simulink model "Continues_motor_control_v9_tensiontest"  (R2025b)
settings: Solver=FixedStepAuto  StartTime=0.0  StopTime=Duration_time  FixedStep=T_sample  RelTol=1e-3  EnableMultiTasking=on
undefined symbols (not defined in the file or in its folder): bias, cyclenum, Ki, Kp, N_finish, N_start, Potent_gain, T, T_sample, v_0, Voltage
libraries: slrealtimeloglib x4, speedgoatlib_IO131 x3, simulink x1
settings Model: Creator=User  LastModifiedBy=paola
settings SolverCC: ConcurrentTasks=on  AlgebraicLoopSolver=TrustRegion  PositivePriorityOrder=on  AutoInsertRateTranBlk=on  InsertRTBMode=Never (minimum delay)
settings DataIOCC: SaveFormat=Array  SaveState=on  SignalLoggingName=logsOut
settings OptimizationCC: BlockReduction=off  BooleanDataType=off  OptimizeBlockIOStorage=off  BufferReuse=off  ReuseModelBlockBuffer=off  GlobalBufferReuse=off  ExpressionFolding=off  LocalBlockOutputs=off  InitFltsAndDblsToZero=on  OptimizeDataStoreBuffers=off  BusAssignmentInplaceUpdate=off
settings DebuggingCC: SaveWithParameterizedLinksMsg=none  UnderspecifiedInitializationDetection=Classic  MergeDetectMultiDrivingBlocksExec=none  CheckExecutionContextPreStartOutputMsg=on  SignalResolutionControl=TryResolveAllWithWarning  TasksWithSamePriorityMsg=none  UnconnectedInputMsg=warning  UnconnectedOutputMsg=warning  UnconnectedLineMsg=warning  SFUnexpectedBacktrackingDiag=warning  SFNoUnconditionalDefaultTransitionDiag=warning  SFExecutionAtInitializationDiag=none  ArithmeticOperatorsInVariantConditions=warning
settings HardwareCC: ProdBitPerLong=64.0  ProdLongLongMode=on  ProdHWDeviceType=Intel->x86-64 (Linux 64)
settings ModelReferenceCC: EnableRefExpFcnMdlSchedulingChecks=on  PropagateSignalLabelsOutOfModel=off
settings SFSimCC: SimUseLocalCustomCode=off  SimTargetLang=C++  SimDLTargetLibrary=mkl-dnn
settings RTWCC: SystemTargetFile=speedgoat.tlc  TemplateMakefile=slrealtime_default_tmf  RTWUseLocalCustomCode=off  Toolchain=Simulink Real-Time Toolchain  BuildConfiguration=Faster Runs  CodeExecutionProfiling=on  TargetLang=C++  GPUComputeCapability=3.5  DLArmComputeVersion=19.05  Description=Speedgoat Real-Time Target Machine
settings CodeAppCC: StateflowObjectComments=on
settings SimulinkRealTimeTargetCC: SLRTFileLogMaxRuns=1.0  ExtModeMaxTrigDuration=10.0  ExtModeStaticAllocSize=1000000.0  ExtModeTransport=0.0  MultiwordLength=2048.0  DynamicStringBufferSize=256.0  PreserveMATLABNamespacesInGeneratedCode=on  SubcomponentCodeInterfacePackaging=Reusable function  InstructionSetFMA=off  LogToMDFFile=off
settings ConfigComp: CovMetricSettings=dw  CovSaveCumulativeToWorkspaceVar=on  CovSaveSingleToWorkspaceVar=on  CovExternalEMLEnable=off  CovSFcnEnable=off

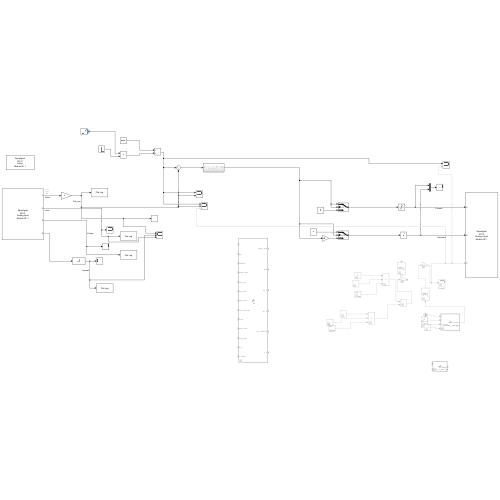
[thumbnail: Simulink's stored preview of the top-level diagram]
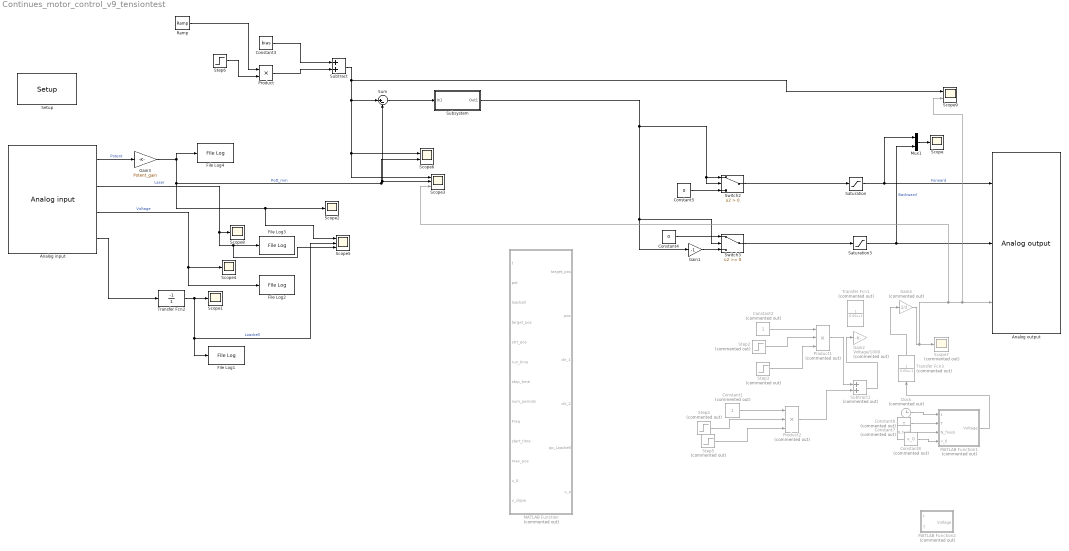
== system Continues_motor_control_v9_tensiontest ==
  "Analog input " : speedgoatlib_IO131/Analog input   parModuleId=1  parSampleTime=-1  parPciSlot=-1  parRange=+-10V  parOversampling=None  parChannels=[1 2 3 4]  parContinuousSampling=off  parDmaEn=off  parDmaChannels=All  parDmaConversionTime=100  parDmaFrameSize=128  parBoardType=131  parIsInitialized=on
      settings: SourceProductName=IO131
  "Analog output " : speedgoatlib_IO131/Analog output   parModuleId=1  parSampleTime=-1  parPciSlot=-1  parRange=+-10V  parChannels=[5 6 7]  parInitValues=[0 0 0]  parResetValues=[1 1 1]  parDmaChannels=All  parDmaEn=off  parDmaClkSrc=2  parDmaConversionTime=100  parDmaFrameSize=128  parBoardType=131  parDoInterrupt=on  parLatency=As small as possible  parIsInitialized=on
      settings: SourceProductName=IO131
  Clock : Clock  Commented=on
  Constant1 : Constant  Commented=on
  Constant2 : Constant  Commented=on
  Constant3 : Constant  Value=bias
  Constant4 : Constant  Value=0
  Constant5 : Constant  Value=0
  Constant6 : Constant  Commented=on  Value=T
  Constant7 : Constant  Commented=on  Value=N_finish
  Constant8 : Constant  Commented=on  Value=v_0
  File Log{1..4} (4 alike) : slrealtimeloglib/File Log  decimation=1  inputProcessing=Elements as channels (sample based)
  Gain1 : Gain  Gain=-1
  Gain2 : Gain  Commented=on  Gain=Voltage/1000
  Gain3 : Gain  Gain=Potent_gain
  Gain4 : Gain  Commented=on  Gain=2/3
  MATLAB Function : MATLAB Function  Commented=on  TreatAsAtomicUnit=on  SystemSampleTime=1/20000
  MATLAB Function1 : MATLAB Function  Commented=on  TreatAsAtomicUnit=on
  MATLAB Function2 : MATLAB Function  Commented=on  TreatAsAtomicUnit=on
  Mux1 : Mux  Inputs=2
  Product : Product
  Product1 : Product  Commented=on  Inputs=3
  Product2 : Product  Commented=on  Inputs=3
  Ramp : simulink/Sources/Ramp  slope=0.5  start=3*T  InitialOutput=0
  Saturation : Saturate  UpperLimit=5  LowerLimit=0
  Saturation3 : Saturate  UpperLimit=5  LowerLimit=0
  Scope{,1..2,4,8} (5 alike) : Scope
      Scope settings: ActiveDisplayYMinimum=-0.62499999999999989  ActiveDisplayYMaximum=5.625
      Scope1 settings: ActiveDisplayYMinimum=-0.40301743822598  ActiveDisplayYMaximum=-0.37430870981834546  DataLoggingVariableName=ScopeData2
      Scope2 settings: ActiveDisplayYMinimum=47.04763  ActiveDisplayYMaximum=48.80097  DataLoggingVariableName=ScopeData3
      Scope4 settings: ActiveDisplayYMinimum=-3.531161659188478  ActiveDisplayYMaximum=3.4859297139005889  DataLoggingVariableName=ScopeData5
      Scope8 settings: ActiveDisplayYMinimum=2.5736629282063022  ActiveDisplayYMaximum=3.1252765697718781  DataLoggingVariableName=ScopeData7
  Scope3 : Scope  NumInputPorts=3
      settings: ActiveDisplayYMinimum=61.500028125  ActiveDisplayYMaximum=146.499996875  DataLoggingVariableName=ScopeData4
  Scope5 : Scope  NumInputPorts=3
      settings: ActiveDisplayYMinimum=34.92623025864043  ActiveDisplayYMaximum=149.50569161516748
  Scope6 : Scope  NumInputPorts=2
      settings: ActiveDisplayYMinimum=-16.874999999999996  ActiveDisplayYMaximum=151.875  DataLoggingVariableName=ScopeData6
  Scope7 : Scope  Commented=on
      settings: ActiveDisplayYMinimum=-4.9999999896942331  ActiveDisplayYMaximum=4.9999999896942331  DataLoggingVariableName=ScopeData2
  Scope9 : Scope  NumInputPorts=2
      settings: ActiveDisplayYMinimum=57.0000140625  ActiveDisplayYMaximum=146.9999984375  DataLoggingVariableName=ScopeData8
  "Setup " : speedgoatlib_IO131/Setup   parPciSlot=-1  parModuleId=1  parTriggerInitiator=Independent  parAdChannels=1:4  parAdRange=+-10V  parAdOversampling=None  parAdContinuousSampling=off  parAdDmaEn=off  parAdDisableCheck=off  parAdDmaChannels=All  parAdSampleClock=1e3  parAdDmaFrameSize=128  parAdSampleTime=-1  parDaChannels=5:7  parDaRange=+-10V  parDaInitValues=0  parDaResetValues=1  parDaDmaEn=off  parDaDisableCheck=off  parDaDmaChannels=All  parLatency=As small as possible  parDaSampleClock=1e3  parClockLocked=on  parDaDmaFrameSize=128  parDaSampleTime=-1  parBoardType=131  parForceRefresh=[]
      settings: SourceProductName=IO131
  Step2 : Step  Commented=on  Time=(N_start-0.25)*T  SampleTime=T_sample
  Step3 : Step  Commented=on  Time=(cyclenum+0.25)*T  Before=1  After=0  SampleTime=T_sample
  Step4 : Step  Commented=on  Time=(2*cyclenum+0.25)*T  SampleTime=T_sample
  Step5 : Step  Commented=on  Time=(cyclenum+0.25)*T  Before=1  After=0  SampleTime=T_sample
  Step6 : Step  Time=N_finish*T  Before=1  After=0  SampleTime=T_sample
  Subsystem : Subsystem
  Subtract : Sum
  Subtract1 : Sum  Commented=on
  Sum : Sum  Inputs=|+-
  Switch2 : Switch  Criteria=u2 > Threshold  SaturateOnIntegerOverflow=off  InputSameDT=off
  Switch3 : Switch  SaturateOnIntegerOverflow=off  InputSameDT=off
  Transfer Fcn1 : TransferFcn  Commented=on  Denominator=[0.05 1]
  Transfer Fcn2 : TransferFcn  Numerator=[-1]  Denominator=[1 ]
  Transfer Fcn3 : TransferFcn  Commented=on  Denominator=[0.05 1]
  wires:
  "Analog input "/4 -> Transfer Fcn2/1
  Constant5/1 -> Switch2/3
  Transfer Fcn2/1 -> Scope5/2, File Log1/1, Scope1/1  "Loadcell"
  Gain3/1 -> Scope6/2, Scope3/2, Sum/2, Scope5/1, Scope2/1, File Log4/1  "Pott_mm"
  Saturation/1 -> "Analog output "/1, Mux1/1  "Forward"
  Gain1/1 -> Switch3/3
  Subsystem/1(Out1) -> Gain1/1, Switch3/2, Switch2/1, Switch2/2
  Constant4/1 -> Switch3/1
  Switch3/1 -> Saturation3/1
  "Analog input "/1 -> Gain3/1  "Potent"
  Sum/1 -> Subsystem/1(In1)
  Mux1/1 -> Scope/1
  Switch2/1 -> Saturation/1
  Saturation3/1 -> "Analog output "/2, Mux1/2  "Backward"
  "Analog input "/3 -> File Log2/1, Scope4/1  "Voltage"
  Step6/1 -> Product/2
  Ramp/1 -> Product/1
  Constant2/1 -> Product1/1
  Transfer Fcn3/1 -> Gain4/1
  Step2/1 -> Product1/2
  Step3/1 -> Product1/3
  Product1/1 -> Subtract1/1
  Product2/1 -> Subtract1/2
  Constant1/1 -> Product2/1
  Step4/1 -> Product2/2
  Step5/1 -> Product2/3
  Subtract1/1 -> Gain2/1
  Clock/1 -> MATLAB Function1/1(t)
  Constant6/1 -> MATLAB Function1/2(T)
  "Analog input "/2 -> Scope5/3, File Log3/1, Scope8/1  "Laser"
  MATLAB Function1/1(Voltage) -> Transfer Fcn3/1
  Product/1 -> Subtract/2
  Constant3/1 -> Subtract/1
  Subtract/1 -> Scope3/1, Scope6/1, Sum/1, Scope9/1
  Gain4/1 -> Scope3/3, Scope9/2, "Analog output "/3, Scope7/1
  Constant7/1 -> MATLAB Function1/3(N_finish)
  Constant8/1 -> MATLAB Function1/4(v_0)

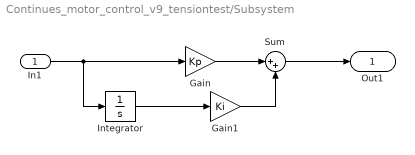
== system Continues_motor_control_v9_tensiontest/Subsystem ==
  In1 : Inport
  Gain : Gain  Gain=Kp
  Gain1 : Gain  Gain=Ki
  Integrator : Integrator
  Sum : Sum  Inputs=|++
  Out1 : Outport
  wires:
  In1/1 -> Integrator/1, Gain/1
  Sum/1 -> Out1/1
  Gain/1 -> Sum/1
  Gain1/1 -> Sum/2
  Integrator/1 -> Gain1/1

== matlab function Continues_motor_control_v9_tensiontest/MATLAB Function1 ==
  data: t input; Voltage output; T input; N_finish input; v_0 input
function Voltage = generate_voltage(t, T, N_finish, v_0)
% Generates a voltage waveform with:
% - 3T initial rest (0 V)
% - N cycles of pattern [0, +2, 0, -2]
% - 1T final rest (0 V)
%
% t : current time
% T : one cycle duration
% N : number of active cycles

   % total_time = Initial a*T rest + applying voltage_time*T + final resting*T;  % total signal duration
     total_time = (N_finish-1)*T;

    if t < 1*T
        % Initial 3T rest
        Voltage = 0;

    elseif t < (1 + (N_finish-2))*T
        % Active part (N cycles)
        active_time = t - 2*T;   % time since the active section started
        phase = mod(active_time, T);
        quarter = T / 4;

        if phase < quarter
            Voltage = 0;
        elseif phase < 2*quarter
            Voltage = v_0;
        elseif phase < 3*quarter
            Voltage = 0;
        elseif phase < 4*quarter
            Voltage = -v_0;
        else
            Voltage = 0;
        end

    elseif t < total_time
        % Final 1T rest
        Voltage = 0;

    else
        % After everything
        Voltage = 0;
    end
end

== matlab function Continues_motor_control_v9_tensiontest/MATLAB Function ==
  data: target_pos output; t input; pot input; loadcell input; pos output; dir_1 output; target_pos input; dir_2 output; strt_pos input; run_time input; stop_time input; num_periods input; Freq input; start_time input; max_pos input; v_0 input; v_slope input; pp_Loadcell output; v_o output
function [target_pos,pos,dir_1,dir_2,pp_Loadcell, v_o] = fcn(t,pot,loadcell,target_pos,strt_pos,run_time,stop_time,num_periods,Freq,start_time,max_pos,v_0,v_slope)

persistent strt_pos_th I;

if isempty(strt_pos_th)
 strt_pos_th = strt_pos;

 I=0;
 last_err=0;
end

v_o=0;
v=0;

loadcell_thr = -0.3; % In N

% cal_loadcell = 2.7384;%0.9936;%-1.6080;
% offset_loadcell =   0.2727; %0.2868;%0.1759;
% 
% cal_weight = 0.399*10;
% pp_Loadcell = (loadcell - offset_loadcell).*(cal_weight/(cal_loadcell-offset_loadcell));
C_1 = 1.5635;
pp_Loadcell = (loadcell-0.3058)*C_1 ;


if(t>(run_time-stop_time))
    v = 0;
elseif(t>(start_time-0.1))
    v = v_0;

    
    if(pp_Loadcell>loadcell_thr)
        target_pos = (strt_pos-3)+5/start_time.*t;
        strt_pos_th = target_pos;
    else
        target_pos = strt_pos_th;
    end

end

%persistent pwm_val;

%if isempty(X)
%  X = [0 0 0]; 
%  P =  diag([10000,10000,10000]);
%end

% if(t>(run_time-stop_time))
%     target_pos=strt_pos-3;
% end

dir_1 = 0;
dir_2 = 0;



v_o=v/1000;

end

== matlab function Continues_motor_control_v9_tensiontest/MATLAB Function2 ==
  data: t input; Voltage output; T input
function Voltage = generate_voltage(t, T)
% t: current time
% T: time period

    if t < (T)
        Voltage = 0;
    elseif t < (T+T*1/4)
        Voltage = 2;
    elseif t < (T+T*1/2)
        Voltage = 0;
    elseif t < (T+T*3/4)
        Voltage = -2;
    elseif t < (2*T)
        Voltage = 0;
    elseif t < (2*T+T*1/4)
        Voltage = 2;
    elseif t < (2*T+T*1/2)
        Voltage = 0;
    elseif t < (2*T+T*3/4)
        Voltage = -2;
    elseif t < (3*T)
        Voltage = 0;
    elseif t < (3*T+T*1/4)
        Voltage = 2;
    elseif t < (3*T+T*1/2)
        Voltage = 0;
    elseif t < (3*T+T*3/4)
        Voltage = -2;
    elseif t < (4*T)
        Voltage = 0;
    elseif t < (4*T+T*1/4)
        Voltage = 2;
    elseif t < (4*T+T*1/2)
        Voltage = 0;
    elseif t < (4*T+T*3/4)
        Voltage = -2;
    elseif t < (5*T)
        Voltage = 0;
    elseif t < (5*T+T*1/4)
        Voltage = 2;
    elseif t < (5*T+T*1/2)
        Voltage = 0;
    elseif t < (5*T+T*3/4)
        Voltage = -2;
    elseif t < (6*T)
        Voltage = 0;
    elseif t < (6*T+T*1/4)
        Voltage = 2; 
    elseif t < (6*T+T*1/2)
        Voltage = 0;
    elseif t < (6*T+T*3/4)
        Voltage = -2;
    elseif t < (7*T)
        Voltage = 0;
    elseif t < (7*T+T*1/4)
        Voltage = 2;
    elseif t < (7*T+T*1/2)
        Voltage = 0;
    elseif t < (7*T+T*3/4)
        Voltage = -2;
    elseif t < (8*T)
        Voltage = 0;
    elseif t < (8*T+T*1/4)
        Voltage = 2;
    elseif t < (8*T+T*1/2)
        Voltage = 0;
    elseif t < (8*T+T*3/4)
        Voltage = -2;
    elseif t < (9*T)
        Voltage = 0;
    elseif t < (9*T+T*1/4)
        Voltage = 2;
    elseif t < (9*T+T*1/2)
        Voltage = 0;
    elseif t < (9*T+T*3/4)
        Voltage = -2;
    elseif t < (10*T)
        Voltage = 0;
    elseif t < (10*T+T*1/4)
        Voltage = 2;
    elseif t < (10*T+T*1/2)
        Voltage = 0;
    elseif t < (10*T+T*3/4)
        Voltage = -2;
    elseif t < (11*T)
        Voltage = 0;
    elseif t < (11*T+T*1/4)
        Voltage = 2;
    elseif t < (11*T+T*1/2)
        Voltage = 0;
    elseif t < (11*T+T*3/4)
        Voltage = -2;
    elseif t < (12*T)
        Voltage = 0;
    elseif t < (12*T+T*1/4)
        Voltage = 2;
    elseif t < (12*T+T*1/2)
        Voltage = 0;
    elseif t < (12*T+T*3/4)
        Voltage = -2;
    elseif t < (13*T)
        Voltage = 0;
    elseif t < (13*T+T*1/4)
        Voltage = 2;
    elseif t < (13*T+T*1/2)
        Voltage = 0;
    elseif t < (13*T+T*3/4)
        Voltage = -2;
    elseif t < (14*T)
        Voltage = 0;
    elseif t < (14*T+T*1/4)
        Voltage = 2;
    elseif t < (14*T+T*1/2)
        Voltage = 0;
    elseif t < (14*T+T*3/4)
        Voltage = -2;
    elseif t < (15*T)
        Voltage = 0;
    elseif t < (15*T+T*1/4)
        Voltage = 2;
    elseif t < (15*T+T*1/2)
        Voltage = 0;
    elseif t < (15*T+T*3/4)
        Voltage = -2;
    elseif t < (16*T)
        Voltage = 0;
    elseif t < (16*T+T*1/4)
        Voltage = 2;
    elseif t < (16*T+T*1/2)
        Voltage = 0;
    elseif t < (16*T+T*3/4)
        Voltage = -2;
    elseif t < (17*T)
        Voltage = 0;
    elseif t < (17*T+T*1/4)
        Voltage = 2;
    elseif t < (17*T+T*1/2)
        Voltage = 0;
    elseif t < (17*T+T*3/4)
        Voltage = -2;
    elseif t < (18*T)
        Voltage = 0;
    elseif t < (18*T+T*1/4)
        Voltage = 2;
    elseif t < (18*T+T*1/2)
        Voltage = 0;
    elseif t < (18*T+T*3/4)
        Voltage = -2;
    elseif t < (19*T)
        Voltage = 0;
    elseif t < (19*T+T*1/4)
        Voltage = 2;
    elseif t < (19*T+T*1/2)
        Voltage = 0;
    elseif t < (19*T+T*3/4)
        Voltage = -2;
        else


        Voltage = 0;
    end
end
